simulink model "Exa1_Fang"  (R2015a)
settings: Solver=ode23t  StartTime=0.0  StopTime=15
settings Model: Creator=victo  LastModifiedBy=victo

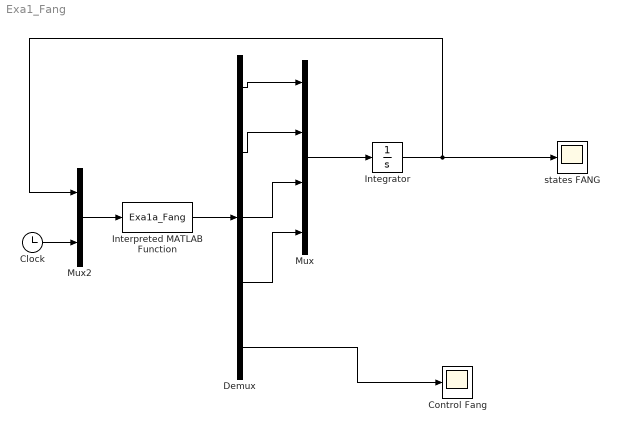
== system Exa1_Fang ==
  Clock : Clock
  Control Fang : Scope
      settings: YMin=-250  YMax=125  SaveName=control_Fang
  Demux : Demux  Outputs=5
  Integrator : Integrator  InitialCondition=[-1.2 0.5 0.7 -0.6]'
  Interpreted MATLAB Function : MATLABFcn  MATLABFcn=Exa1a_Fang  OutputDimensions=5
  Mux : Mux
  Mux2 : Mux  Inputs=2
  states FANG : Scope
      settings: TimeRange=10  YMin=-0.4  YMax=0.4  SaveName=todos
  wires:
  Integrator/1 -> Mux2/1, states FANG/1
  Interpreted MATLAB Function/1 -> Demux/1
  Mux/1 -> Integrator/1
  Demux/2 -> Mux/2
  Demux/1 -> Mux/1
  Mux2/1 -> Interpreted MATLAB Function/1
  Clock/1 -> Mux2/2
  Demux/3 -> Mux/3
  Demux/4 -> Mux/4
  Demux/5 -> Control Fang/1
